simulink model "HeatExch1_sf_sim"  (R2017a)
settings: Solver=VariableStepAuto  StartTime=0.0  StopTime=6367  RelTol=1e-3
settings Model: Creator=eliwi  LastModifiedBy=eliwi

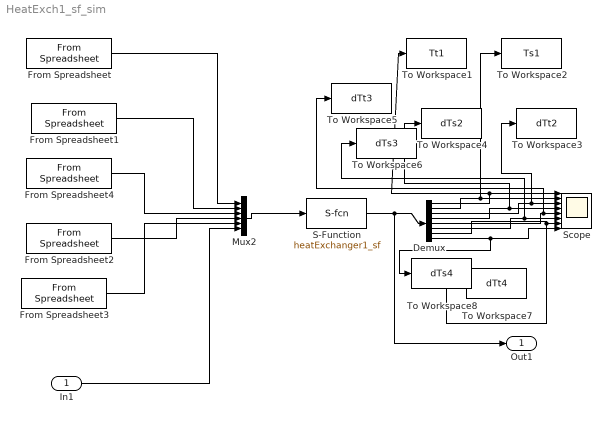
== system HeatExch1_sf_sim ==
  In1 : Inport
  Demux : Demux  Outputs=8
  From Spreadsheet : FromSpreadsheet  FileName=Day2.xlsx  SheetName=T3
  From Spreadsheet1 : FromSpreadsheet  FileName=Day2.xlsx  SheetName=T4
  From Spreadsheet2 : FromSpreadsheet  FileName=Day2.xlsx  SheetName=Ft
  From Spreadsheet3 : FromSpreadsheet  FileName=Day2.xlsx  SheetName=Fs
  From Spreadsheet4 : FromSpreadsheet  FileName=Day2.xlsx  SheetName=T6
  Mux2 : Mux  Inputs=6
  S-Function : S-Function  FunctionName=heatExchanger1_sf  SFunctionDeploymentMode=off  EnableBusSupport=off
  Scope : Scope  NumInputPorts=8
  To Workspace1 : ToWorkspace  VariableName=Tt1  SaveFormat=Timeseries  SampleTime=-1
  To Workspace2 : ToWorkspace  VariableName=Ts1  SaveFormat=Timeseries  SampleTime=-1
  To Workspace3 : ToWorkspace  VariableName=dTt2  SaveFormat=Timeseries  SampleTime=-1
  To Workspace4 : ToWorkspace  VariableName=dTs2  SaveFormat=Timeseries  SampleTime=-1
  To Workspace5 : ToWorkspace  VariableName=dTt3  SaveFormat=Timeseries  SampleTime=-1
  To Workspace6 : ToWorkspace  VariableName=dTs3  SaveFormat=Timeseries  SampleTime=-1
  To Workspace7 : ToWorkspace  VariableName=dTt4  SaveFormat=Timeseries  SampleTime=-1
  To Workspace8 : ToWorkspace  VariableName=dTs4  SaveFormat=Timeseries  SampleTime=-1
  Out1 : Outport
  wires:
  S-Function/1 -> Out1/1, Demux/1
  Mux2/1 -> S-Function/1
  From Spreadsheet/1 -> Mux2/1
  From Spreadsheet1/1 -> Mux2/2
  From Spreadsheet4/1 -> Mux2/3
  From Spreadsheet2/1 -> Mux2/4
  From Spreadsheet3/1 -> Mux2/5
  In1/1 -> Mux2/6
  Demux/2 -> To Workspace2/1, Scope/2
  Demux/3 -> To Workspace3/1, Scope/3
  Demux/4 -> To Workspace4/1, Scope/4
  Demux/5 -> To Workspace5/1, Scope/5
  Demux/6 -> To Workspace6/1, Scope/6
  Demux/7 -> To Workspace7/1, Scope/7
  Demux/8 -> To Workspace8/1, Scope/8
  Demux/1 -> Scope/1, To Workspace1/1
